simulink model "pendule_inv_capteur_etu"  (R2017a)
settings: Solver=VariableStepAuto  StartTime=0.0  StopTime=10.0  RelTol=1e-3
values from neighbouring files (symbols this model uses):
  K = [30 10]    [exemple_test_pendule_inv.m]
  ue = 0    [exemple_test_pendule_inv.m]
  x0 = [pi/10 0]    [exemple_test_pendule_inv.m]
  xe = [0 0]    [exemple_test_pendule_inv.m]
settings Model: Creator=jky  LastModifiedBy=jky

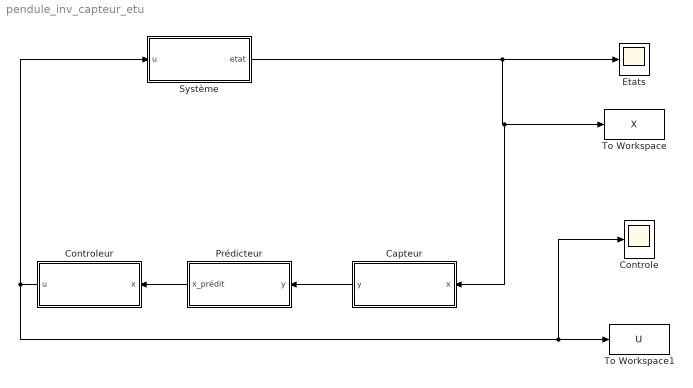
== system pendule_inv_capteur_etu ==
  Capteur : Subsystem
  Controle : Scope
  Controleur : Subsystem
  Etats : Scope
  Prédicteur : Subsystem
  Système : Subsystem
  To Workspace : ToWorkspace  VariableName=X  SaveFormat=Timeseries  SampleTime=-1
  To Workspace1 : ToWorkspace  VariableName=U  SaveFormat=Timeseries  SampleTime=-1
  wires:
  Système/1(etat) -> Capteur/1(x), To Workspace/1, Etats/1
  Prédicteur/1("x_prédit ") -> Controleur/1(x)
  Capteur/1(y) -> Prédicteur/1(y)
  Controleur/1(u) -> Système/1(u), Controle/1, To Workspace1/1

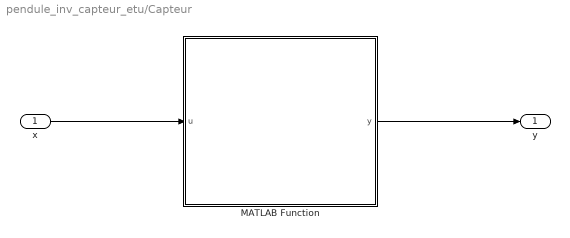
== system pendule_inv_capteur_etu/Capteur ==
  x : Inport
  MATLAB Function : MATLAB Function  TreatAsAtomicUnit=on
  y : Outport
  wires:
  x/1 -> MATLAB Function/1(u)
  MATLAB Function/1(y) -> y/1

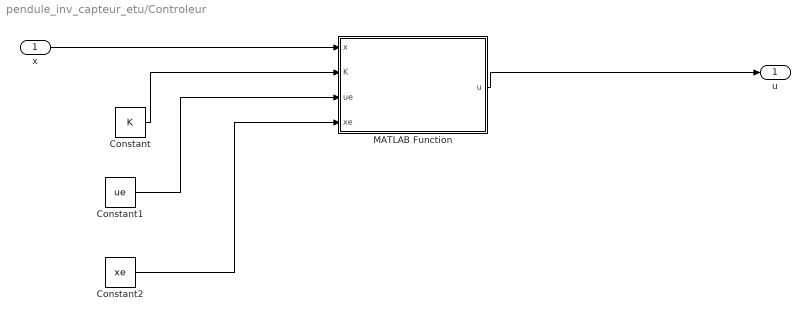
== system pendule_inv_capteur_etu/Controleur ==
  x : Inport
  Constant : Constant  Value=K
  Constant1 : Constant  Value=ue
  Constant2 : Constant  Value=xe
  MATLAB Function : MATLAB Function  TreatAsAtomicUnit=on
  u : Outport
  wires:
  x/1 -> MATLAB Function/1(x)
  MATLAB Function/1(u) -> u/1
  Constant/1 -> MATLAB Function/2(K)
  Constant1/1 -> MATLAB Function/3(ue)
  Constant2/1 -> MATLAB Function/4(xe)

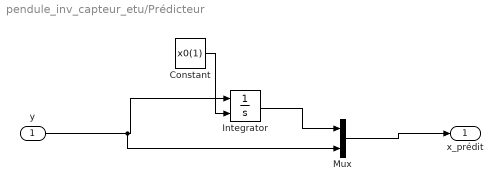
== system pendule_inv_capteur_etu/Prédicteur ==
  y : Inport
  Constant : Constant  Value=x0(1)
  Integrator : Integrator  InitialConditionSource=external
  Mux : Mux  Inputs=2
  "x_prédit " : Outport
  wires:
  Integrator/1 -> Mux/1
  Mux/1 -> "x_prédit "/1
  Constant/1 -> Integrator/2
  y/1 -> Mux/2, Integrator/1

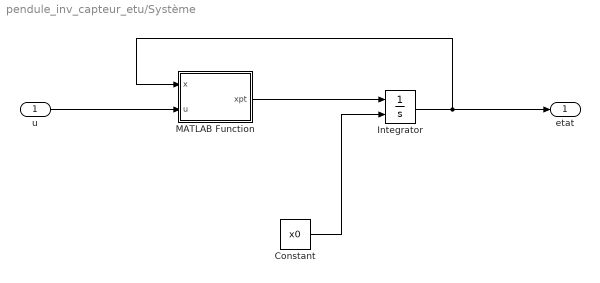
== system pendule_inv_capteur_etu/Système ==
  u : Inport
  Constant : Constant  Value=x0
  Integrator : Integrator  InitialConditionSource=external  InitialCondition=[pi/20 0]
  MATLAB Function : MATLAB Function  TreatAsAtomicUnit=on
  etat : Outport
  wires:
  Constant/1 -> Integrator/2
  u/1 -> MATLAB Function/2(u)
  Integrator/1 -> etat/1, MATLAB Function/1(x)
  MATLAB Function/1(xpt) -> Integrator/1

== matlab function pendule_inv_capteur_etu/Controleur/MATLAB Function ==
  data: x input; u output; K input; ue input; xe input
function u = fcn(x, K, ue, xe)
u = ue + K(:)'*(x(:)-xe);

== matlab function pendule_inv_capteur_etu/Système/MATLAB Function ==
  data: x input; u input; xpt output
function xpt = fcn(x,u)
g = 9.81;
l = 10;
xpt = transpose([x(2) ((g/l)*sin(x(1)))-((cos(x(1))*u)/l)]);

== matlab function pendule_inv_capteur_etu/Capteur/MATLAB Function ==
  data: u input; y output
function y = fcn(u)

y = u(2);
